simulink model "power_2machinesSVC_PSS"  (Simulink 6.0)
settings: Solver=ode23tb  StartTime=0.0  StopTime=50  MaxStep=1/60  RelTol=1e-4  AbsTol=1e-3
undefined symbols (not defined in the file or in its folder): D1, Delta, find_system, j
libraries: powerlib x18, powerlib2 x8, powerlib_extras x4, simulink_extras x1
settings Model: Creator=sybille  LastModifiedBy=batserve  ExtModeTrigMode=oneshot  ExtModeArmWhenConnect=off  ExtModeAutoUpdateStatusClock=off
settings DataIOCC: LimitDataPoints=off  SignalLoggingName=sigsOut
settings OptimizationCC: BlockReduction=off  BooleanDataType=off
settings DebuggingCC: SolverPrmCheckMsg=none
settings HardwareCC: TargetUnknown=on

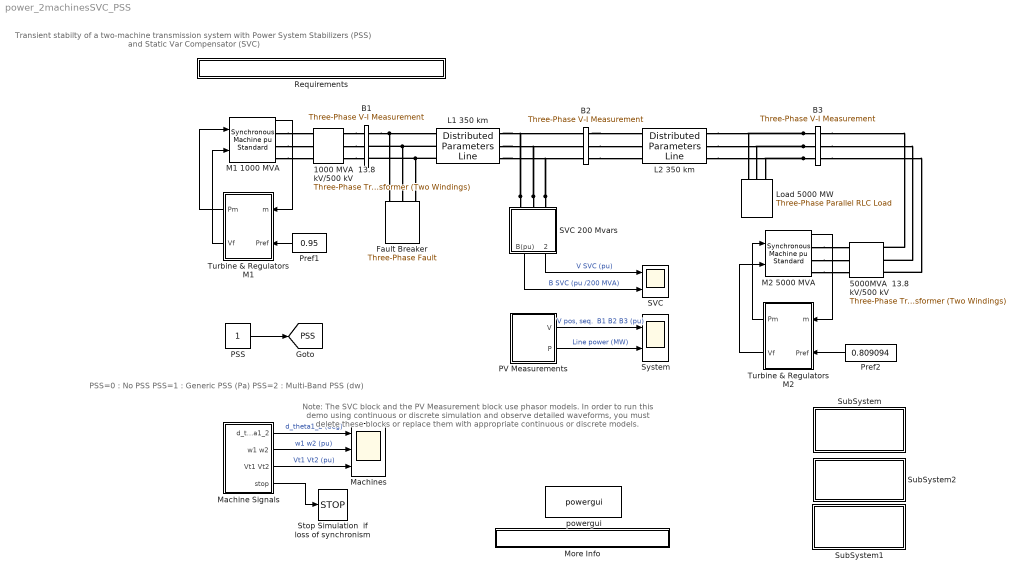
== system power_2machinesSVC_PSS ==
  note: Transient stabilty of a two-machine transmission system
      | with Power System Stabilizers (PSS) and Static Var Compensator (SVC)
  note: Note:
      | The SVC block and the PV Measurement block
      | use phasor models.  In order to run this demo using
      | continuous or discrete simulation and observe detailed
      | waveforms,  you must delete these blocks or replace
      | them with appropriate continuous or discrete models.
  note: PSS=0 : No PSS
      | PSS=1 : Generic PSS (Pa)
      | PSS=2 : Multi-Band PSS (dw)
  1000 MVA  13.8 kV/500 kV : powerlib/Elements/Three-Phase Transformer (Two Windings)  NominalPower=[ 1000e6 60 ]  Winding1Connection=Delta (D1)  Winding1="[ 13.8e3 0.002  0.0]"  Winding2Connection=Yg  Winding2=[ 500e3 0.002 0.12]  SetSaturation=off  Rm=500  Lm=500  Saturation="[ 0,0  ;  0.005,1.2  ;  1.0,1.4 ]"  Hysteresis=off  DataFile='hysteresis'  SetInitialFlux=off  InitialFluxes=[ 0.8 , -0.8 , 0.7 ]  Measurements=None  TransfoNumber=0
  5000MVA  13.8 kV/500 kV : powerlib/Elements/Three-Phase Transformer (Two Windings)  NominalPower=[ 5000e6 60 ]  Winding1Connection=Delta (D1)  Winding1="[ 13.8e3 0.002  0.0]"  Winding2Connection=Yg  Winding2=[ 500e3 0.002 0.12]  SetSaturation=off  Rm=500  Lm=500  Saturation="[ 0,0  ;  0.005,1.2  ;  1.0,1.4 ]"  Hysteresis=off  DataFile='hysteresis'  SetInitialFlux=off  InitialFluxes=[ 0.8 , -0.8 , 0.7 ]  Measurements=None  TransfoNumber=0
  B1 : powerlib/Measurements/Three-Phase V-I Measurement  VoltageMeasurement=phase-to-ground  SetLabelV=on  LabelV=Vabc_B1  Vpu=on  Vbase=500e3  CurrentMeasurement=yes  SetLabelI=on  LabelI=Iabc_B1  Ipu=on  Pbase=100e6  OutputType=Complex  PhasorSimulation=on  PSBequivalent=0
  B2 : powerlib/Measurements/Three-Phase V-I Measurement  VoltageMeasurement=phase-to-ground  SetLabelV=on  LabelV=Vabc_B2  Vpu=on  Vbase=500e3  CurrentMeasurement=no  SetLabelI=on  LabelI=Iabc_B2  Ipu=on  Pbase=100e6  OutputType=Complex  PhasorSimulation=on  PSBequivalent=0
  B3 : powerlib/Measurements/Three-Phase V-I Measurement  VoltageMeasurement=phase-to-ground  SetLabelV=on  LabelV=Vabc_B3  Vpu=on  Vbase=500e3  CurrentMeasurement=no  SetLabelI=off  LabelI=I1  Ipu=off  Pbase=0  OutputType=Complex  PhasorSimulation=on  PSBequivalent=0
  Fault Breaker : powerlib/Elements/Three-Phase Fault  Orientation=down  FaultA=on  FaultB=off  FaultC=off  FaultResistance=0.001  GroundFault=on  GroundResistance=0.001  External=off  SwitchStatus=[1 0]  SwitchTimes=[ 0.1 0.2]  InitialStates=[0 0 1]  SnubberResistance=1e6  SnubberCapacitance=inf  Measurements=None
  L1 350 km : powerlib/Elements/Distributed Parameters Line  Phases=3  Frequency=60  Resistance="[0.01755  0.2758]"  Inductance="[0.8737e-3  3.220e-3]"  Capacitance="[13.33e-9  8.297e-9]"  Length=350  x1=[0 -2.08119625850685e-008 487443.70964158 -112421.385718226;0.000361814960995258 -1.32408804911861e-008 498203.083338567 -45095.3864412803;0.000723629921990516 -5.4238303493389e-009 499707.631423288 23068.3233023193;0.00108544488298577 2.49397509835117e-009 491929.404791019 90803.5063738243;0.00144725984398103 1.03654514377148e-008 475012.894982382 156851.886122394;0.00180907480497629 1.80443748831749e-008 449272.350048993 219986.520650259]  x2=[0 -2.35529805500378e-008 400923.037995999 -306678.651465529;0.000361814960995258 -1.81656675870373e-008 438900.84018104 -249313.294277769;0.000723629921990516 -1.2440901703188e-008 468725.439640532 -187316.590680232;0.00108544488298577 -6.48502850673286e-009 489842.802334574 -121840.216966217;0.00144725984398103 -4.08686750512464e-010 501860.643438643 -54100.489213872;0.00180907480497629 5.67524693906307e-009 504555.714588018 14644.2315021005]  x3=[0 -2.28639731612497e-011 13.1153359399388 -184.480419316447;0.000361814960995258 -1.5497855368557e-011 38.0787449775036 -180.983668896994;0.000723629921990516 -7.84384303326341e-012 62.3347875693628 -174.124891323704;0.00108544488298577 -4.41202400649915e-014 85.4328734808534 -164.031498072894;0.00144725984398103 7.75642214887949e-012 106.943923157398 -150.890988173566;0.00180907480497629 1.54128780462632e-011 126.468338482985 -134.947465148244]  x4=[0 -8.91581395814244e-011 3023.50620810601 -2208.10451815775;0.000361814960995258 -8.08885983149858e-011 3295.677846705 -1776.46366568912;0.000723629921990516 -7.11164371401972e-011 3506.62761662129 -1311.82249270399;0.00108544488298577 -6.00231877467494e-011 3652.43682806992 -822.812364948711;0.00144725984398103 -4.7814922903044e-011 3730.39686910176 -318.517335907422;0.00180907480497629 -3.47184283635963e-011 3739.05952189439 191.694602315866]  x5=0.00180907480497629  Measurements=None
      settings: AttributesFormatString=\n
  L2 350 km : powerlib/Elements/Distributed Parameters Line  Phases=3  Frequency=60  Resistance="[0.01755  0.2758]"  Inductance="[0.8737e-3  3.220e-3]"  Capacitance="[13.33e-9  8.297e-9]"  Length=350  x1=[0 -2.35529805500378e-008 400923.037995999 -306678.651465529;0.000361814960995258 -1.81656675870373e-008 438900.84018104 -249313.294277769;0.000723629921990516 -1.2440901703188e-008 468725.439640532 -187316.590680232;0.00108544488298577 -6.48502850673286e-009 489842.802334574 -121840.216966217;0.00144725984398103 -4.08686750512464e-010 501860.643438643 -54100.489213872;0.00180907480497629 5.67524693906307e-009 504555.714588018 14644.2315021005]  x2=[0 -1.22208025570452e-008 237673.529594385 -435607.401325092;0.000361814960995258 -1.12033805949038e-008 294699.1687201 -399242.932774381;0.000723629921990516 -9.97784002181595e-009 346250.354744666 -355461.963115335;0.00108544488298577 -8.56694698408616e-009 391369.451610182 -305077.785667245;0.00144725984398103 -6.9969108117215e-009 429218.308395391 -249026.357656179;0.00180907480497629 -5.29689714312553e-009 459093.829152304 -188348.913488164]  x3=[0 2.19231358823738e-011 52.7160632692662 -144.994726298769;0.000361814960995258 2.8947525098237e-011 71.9423984147416 -136.479806556214;0.000723629921990516 3.54341731686708e-011 89.8323019448307 -125.429581731223;0.00108544488298577 4.12625814482279e-011 106.053443645353 -112.049325350098;0.00144725984398103 4.63244790248479e-011 120.30449290899 -96.5875945647238;0.00180907480497629 5.05258340049004e-011 132.320716376721 -79.3316128525696]  x4=[0 -9.73737691565742e-011 1740.3123490764 -3266.29894983194;0.000361814960995258 -9.76379763309758e-011 2168.29428893824 -2999.31609805074;0.000723629921990516 -9.60884202544106e-011 2555.99710128903 -2676.61671545742;0.00108544488298577 -9.275388611859e-011 2896.21865904908 -2304.19539865519;0.00144725984398103 -8.76963176026223e-011 3182.63886647449 -1888.97039937023;0.00180907480497629 -8.10096661817247e-011 3409.93706385801 -1438.65510815903]  x5=0.00180907480497629  Measurements=None
      settings: AttributesFormatString=\n
  Load 5000 MW : powerlib/Elements/Three-Phase Parallel RLC Load  Orientation=down  PhysicalDomain=powersysdomain  SubClassName=unknown  LeftPortType=p1  RightPortType=p1  LConnTagsString=A|B|C  Configuration=Y (grounded)  NominalVoltage=500e3  NominalFrequency=60  ActivePower=5000e6  InductivePower=0  CapacitivePower=0  Measurements=None
  M1 1000 MVA : powerlib/Machines/Synchronous Machine pu Standard  PresetModel=No  ShowDetailedParameters=on  RotorType=Salient-pole  NominalParameters="[1000E6  13800   60 ]"  Reactances1=[ 31 32 33 34 35 36 37 ]  Reactances2=[ 1.305, 0.296, 0.252, 0.474, 0.243, 0.18 ]  dAxisTimeConstants=Short-circuit  qAxisTimeConstants=Open-circuit  TimeConstants1=[]  TimeConstants2=[]  TimeConstants3=[]  TimeConstants4=[]  TimeConstants5=[ 1.01, 0.053, 0.1 ]  TimeConstants6=[]  TimeConstants7=[]  TimeConstants8=[]  StatorResistance=2.8544e-3  Mechanical="[ 3.7 0  32]"  InitialConditions=[0 -16.6861 0.950218 0.950218 0.950218 48.1093 -71.8907 168.109 1.44424]  SetSaturation=off  Saturation=[0.6404,0.7127,0.8441,0.9214,0.9956,1.082,1.19,1.316,1.457;0.7,0.7698,0.8872,0.9466,0.9969,1.046,1.1,1.151,1.201]  Units=0.5  LoadFlowParameters=[1 950000000 0 0]
      settings: AttributesFormatString=\n\n
  M2 5000 MVA : powerlib/Machines/Synchronous Machine pu Standard  PresetModel=No  ShowDetailedParameters=on  RotorType=Salient-pole  NominalParameters="[5000E6  13800   60 ]"  Reactances1=[ 31 32 33 34 35 36 37 ]  Reactances2=[ 1.305, 0.296, 0.252, 0.474, 0.243, 0.18 ]  dAxisTimeConstants=Short-circuit  qAxisTimeConstants=Open-circuit  TimeConstants1=[]  TimeConstants2=[]  TimeConstants3=[]  TimeConstants4=[]  TimeConstants5=[ 1.01, 0.053, 0.1 ]  TimeConstants6=[]  TimeConstants7=[]  TimeConstants8=[]  StatorResistance=2.8544e-3  Mechanical="[ 3.7 0  32]"  InitialConditions=[0 -69.7487 0.812764 0.812764 0.812764 -5.44703 -125.447 114.553 1.40021]  SetSaturation=off  Saturation=[0.6404,0.7127,0.8441,0.9214,0.9956,1.082,1.19,1.316,1.457;0.7,0.7698,0.8872,0.9466,0.9969,1.046,1.1,1.151,1.201]  Units=0.5  LoadFlowParameters=[2 4000000000 0 0]
      settings: AttributesFormatString=\n\n
  Machine Signals : Subsystem
  Machines : Scope  NumInputPorts=3
      settings: TimeRange=50  YMin=30~0.995~0  YMax=70~1.005~1.5  SaveName=mach
  More Info : Subsystem
      settings: OpenFcn=web(which('psb2machines.html'));
      mask Display: disp('? : Double click here for more info')
  PSS : Constant
  PV Measurements : Subsystem
  "Pref1 " : Constant  Orientation=left  Value=0.95
  Pref2 : Constant  Orientation=left  Value=0.809094
  Requirements : Subsystem  Description=|  LoadFcn=|  InitFcn=|
      LoadFcn=|
      | Toolboxes = ver;                                                                                                                              
      | installedtoolboxes = {Toolboxes.Name};                                                                                                        
      | k = strcmp('Control System Toolbox',installedtoolboxes);                                                                                      
      | if ~any(k)                                                                                                                                    
      |     H = warndlg(['You need to install the Control System Toolbox in order to run the power_2machinesSVC_PSS demo'],'SimPowerSystems warning');
      |     uiwait(H);                                                                                                                                
      | end
      InitFcn=|
      | Toolboxes = ver;                                                                                               
      | installedtoolboxes = {Toolboxes.Name};                                                                         
      | k = strcmp('Control System Toolbox',installedtoolboxes);                                                       
      | if ~any(k)                                                                                                     
      |     error(['You need to install the Control System Toolbox in order to run the power_2machinesSVC_PSS demo.']);
      | end
      Description=|
      | This block is used to popup errors and warnings if the
      | Control System Toolbox is not installed.
      settings: OpenFcn=|
      | Toolboxes = ver;
      | installedtoolboxes = {Toolboxes.Name};
      | k = strcmp('Control System Toolbox',installedtoolboxes);
      | if ~any(k)
      |     warndlg(['You need to install the Control System Toolbox in order to run the power_2machinesSVC_PSS demo.'],'SimPowerSystems warning');
      |                                                                                                                                                         end
      mask Display: disp('This demo requires the Control System Toolbox')
  SVC : Scope  NumInputPorts=2
      settings: TimeRange=10  YMin=0.5~-1  YMax=1.1~1  SaveName=svc
  SVC 200 Mvars : Subsystem  Orientation=down  AncestorBlock=powerlib/Phasor Elements/Static Var Compensator  LoadFcn=find_system(gcs,'FollowLinks', 'on', 'LookUnderMasks', 'all');  mask(Static Var Compensator (Phasor Type)){mode=Var control (Fixed susceptance Bref), Vnom=500e3, Qnom=[200e6 -200e6], Pbase=200e6, Vref=1.009, Xs=0.03, Kp_Ki=[0  333], Bref=0.0, Tm=8e-3, Td=4e-3}
      mask prompts: mode "Mode of operation"; Vnom "Nominal voltage (Vrms Ph-Ph):"; Qnom "Reactive power limits [Qc(var>0)  Ql(var<0)]:"; Pbase "Three-phase base power Pbase (VA):"; Vref "Reference voltage Vref  (pu):"; Xs "Droop Xs (pu/Pbase):"; Kp_Ki "Voltage regulator [Kp(puB/puV)  Ki(puB/puV/s)]:"; Bref "Bref  for var control mode (pu/Pbase):"; Tm "Time constant of voltage measurement system Tm (s):"; Td "Average time delay due to thyristor valves firing Td (s):"
      mask help:
      | This block implements a  phasor model of a three-phase, three-wire Static Var Compensator (SVC).
      |
      | The B output signal (SVC susceptance in pu/Pbase)  is the output of the voltage regulator or the reference susceptance Bref in var control mode.
      | The Vm output is the measured positive-sequence voltage (pu).
      mask init:
      | Qc_nom=Qnom(1);
      | Ql_nom=Qnom(2);
      | Bmax=Qc_nom/Pbase;
      | Bmin=Ql_nom/Pbase;
      | Vbase=Vnom/sqrt(3)*sqrt(2);
      | Ibase=Pbase/Vnom/sqrt(3)*sqrt(2);
      | Kp=Kp_Ki(1);
      | Ki=Kp_Ki(2);;
      settings: CloseFcn=%3phaseVImeasurement
      mask Help: web(psbhelp)
      mask StyleString: popup(Voltage regulation|Var control (Fixed susceptance Bref)),edit,edit,edit,edit,edit,edit,edit,edit,edit
      mask CallbackString: powericon('psbcallbacks',gcb,'SVCblock');|||||||||
  Stop Simulation  if loss of synchronism : Stop
  SubSystem : Subsystem
      settings: OpenFcn=openfig('psb2macSVC_PhasorVsDet.fig');
      mask Display: disp('Show comparison\nDetailed vs Phasor\n simulation')
  SubSystem1 : Subsystem
      settings: OpenFcn=openfig('psb2macSVC_3phfault.fig');
      mask Display: disp('Show impact of SVC\nfor 3-phase fault')
  SubSystem2 : Subsystem
      settings: OpenFcn=openfig('psb2macSVC_1phfault.fig');
      mask Display: disp('Show impact of PSS\nfor 1-phase fault')
  System : Scope  NumInputPorts=2
      settings: TimeRange=50  YMin=0~0  YMax=1.5~1500  SaveName=mach1
  Turbine & Regulators M1 : Subsystem  Orientation=left
  Turbine & Regulators M2 : Subsystem  Orientation=left
  powergui : powerlib/powergui  Priority=2  Frange=[0:2:500]  Ylog=off  Xlog=off  save=off  variable=ZData  ZoomFFT=on  StartTime=0.0  cycles=1  DisplayStyle=off  fundamental=60  FreqAxis=off  MaxFrequency=1000  frequencyindice=60  frequencyindicesteady=1  RmsSteady=1  display=off  Ts=0  methode=on  frequency=60  echomessages=on
  tag scope: PSS=global
  wires:
  Pref2/1 -> Turbine & Regulators M2/2(Pref)
  Machine Signals/2(w1 w2) -> Machines/2  "w1 w2 (pu)"
  Machine Signals/1(d_theta1_2) -> Machines/1  "d_theta1_2 (deg)"
  Machine Signals/4(stop) -> Stop Simulation  if loss of synchronism/1
  Machine Signals/3(Vt1 Vt2) -> Machines/3  "Vt1 Vt2 (pu)"
  "Pref1 "/1 -> Turbine & Regulators M1/2(Pref)
  PV Measurements/1(V) -> System/1  "V pos, seq.  B1 B2 B3 (pu)"
  PV Measurements/2(P) -> System/2  "Line power (MW)"
  Turbine & Regulators M1/1(Pm) -> M1 1000 MVA/1
  Turbine & Regulators M1/2(Vf) -> M1 1000 MVA/2
  SVC 200 Mvars/2(Vm(pu)) -> SVC/1  "V SVC (pu)"
  SVC 200 Mvars/1(B(pu)) -> SVC/2  "B SVC (pu /200 MVA)"
  Turbine & Regulators M2/1(Pm) -> M2 5000 MVA/1
  Turbine & Regulators M2/2(Vf) -> M2 5000 MVA/2
  M1 1000 MVA/1 -> Turbine & Regulators M1/1(m)
  M2 5000 MVA/1 -> Turbine & Regulators M2/1(m)
  PSS/1 -> [PSS]
  connections:
  B3/LConn3 -- L2 350 km/RConn3 -- Load 5000 MW/LConn3
  B3/LConn2 -- L2 350 km/RConn2 -- Load 5000 MW/LConn2
  B3/LConn1 -- L2 350 km/RConn1 -- Load 5000 MW/LConn1
  L1 350 km/LConn2 -- B1/RConn2 -- Fault Breaker/LConn2
  1000 MVA  13.8 kV/500 kV/RConn2 -- B1/LConn2
  1000 MVA  13.8 kV/500 kV/RConn1 -- B1/LConn1
  L1 350 km/LConn3 -- B1/RConn3 -- Fault Breaker/LConn3
  1000 MVA  13.8 kV/500 kV/RConn3 -- B1/LConn3
  M1 1000 MVA/RConn1 -- 1000 MVA  13.8 kV/500 kV/LConn1
  M1 1000 MVA/RConn2 -- 1000 MVA  13.8 kV/500 kV/LConn2
  M1 1000 MVA/RConn3 -- 1000 MVA  13.8 kV/500 kV/LConn3
  M2 5000 MVA/RConn1 -- 5000MVA  13.8 kV/500 kV/LConn1
  M2 5000 MVA/RConn2 -- 5000MVA  13.8 kV/500 kV/LConn2
  M2 5000 MVA/RConn3 -- 5000MVA  13.8 kV/500 kV/LConn3
  SVC 200 Mvars/LConn2 -- L1 350 km/RConn2 -- B2/LConn2
  SVC 200 Mvars/LConn1 -- L1 350 km/RConn1 -- B2/LConn1
  SVC 200 Mvars/LConn3 -- L1 350 km/RConn3 -- B2/LConn3
  B2/RConn1 -- L2 350 km/LConn1
  B2/RConn2 -- L2 350 km/LConn2
  B2/RConn3 -- L2 350 km/LConn3
  B1/RConn1 -- L1 350 km/LConn1 -- Fault Breaker/LConn1
  B3/RConn1 -- 5000MVA  13.8 kV/500 kV/RConn1
  B3/RConn2 -- 5000MVA  13.8 kV/500 kV/RConn2
  B3/RConn3 -- 5000MVA  13.8 kV/500 kV/RConn3

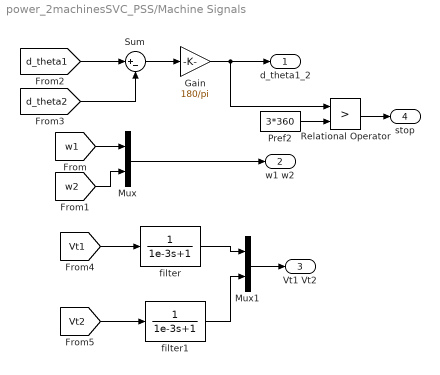
== system power_2machinesSVC_PSS/Machine Signals ==
  " filter" : TransferFcn  Denominator=[1e-3 1]
  " filter1" : TransferFcn  Denominator=[1e-3 1]
  Gain : Gain  Gain=180/pi  SaturateOnIntegerOverflow=on
  Mux : Mux  Inputs=2
  Mux1 : Mux  Inputs=2
  Pref2 : Constant  Value=3*360
  Relational Operator : RelationalOperator  Operator=>  InputSameDT=on
  Sum : Sum  Inputs=|+-  SaturateOnIntegerOverflow=on  InputSameDT=on
  d_theta1_2 : Outport
  w1 w2 : Outport  Port=2
  Vt1 Vt2 : Outport  Port=3
  stop : Outport  Port=4
  wires:
  Sum/1 -> Gain/1
  [d_theta1] -> Sum/1
  [w1] -> Mux/1
  Mux/1 -> w1 w2/1
  Gain/1 -> d_theta1_2/1, Relational Operator/1
  [w2] -> Mux/2
  [d_theta2] -> Sum/2
  [Vt1] -> " filter"/1
  Mux1/1 -> Vt1 Vt2/1
  [Vt2] -> " filter1"/1
  Pref2/1 -> Relational Operator/2
  Relational Operator/1 -> stop/1
  " filter"/1 -> Mux1/1
  " filter1"/1 -> Mux1/2

== system power_2machinesSVC_PSS/More Info ==

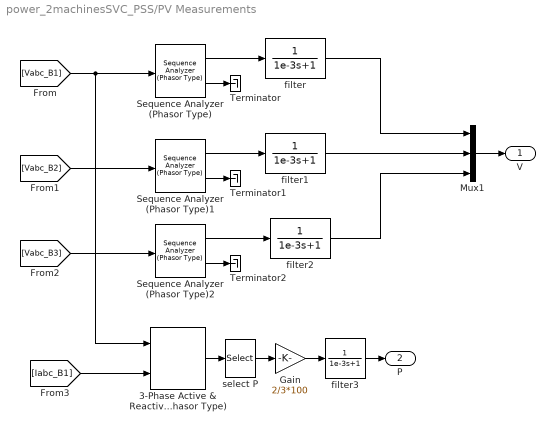
== system power_2machinesSVC_PSS/PV Measurements ==
   filter{,1..3} (4 alike) : TransferFcn  Denominator=[1e-3 1]
  3-Phase Active & Reactive Power (Phasor Type) : powerlib_extras/Phasor Library/3-Phase Active & Reactive Power (Phasor Type)
  Gain : Gain  Gain=2/3*100  SaturateOnIntegerOverflow=on
  Mux1 : Mux  Inputs=3
  Sequence Analyzer (Phasor Type) : powerlib_extras/Phasor Library/Sequence Analyzer (Phasor Type)  seq=Positive
  Sequence Analyzer (Phasor Type)1 : powerlib_extras/Phasor Library/Sequence Analyzer (Phasor Type)  seq=Positive
  Sequence Analyzer (Phasor Type)2 : powerlib_extras/Phasor Library/Sequence Analyzer (Phasor Type)  seq=Positive
  Terminator : Terminator
  Terminator1 : Terminator
  Terminator2 : Terminator
  select P : Selector  InputPortWidth=2
  V : Outport
  P : Outport  Port=2
  wires:
  " filter3"/1 -> P/1
  Gain/1 -> " filter3"/1
  3-Phase Active & Reactive Power (Phasor Type)/1 -> select P/1
  [Iabc_B1] -> 3-Phase Active & Reactive Power (Phasor Type)/2
  Sequence Analyzer (Phasor Type)2/2 -> Terminator2/1
  Sequence Analyzer (Phasor Type)1/2 -> Terminator1/1
  Sequence Analyzer (Phasor Type)/2 -> Terminator/1
  " filter2"/1 -> Mux1/3
  " filter1"/1 -> Mux1/2
  " filter"/1 -> Mux1/1
  Mux1/1 -> V/1
  Sequence Analyzer (Phasor Type)2/1 -> " filter2"/1
  Sequence Analyzer (Phasor Type)1/1 -> " filter1"/1
  [Vabc_B3] -> Sequence Analyzer (Phasor Type)2/1
  [Vabc_B2] -> Sequence Analyzer (Phasor Type)1/1
  Sequence Analyzer (Phasor Type)/1 -> " filter"/1
  [Vabc_B1] -> 3-Phase Active & Reactive Power (Phasor Type)/1, Sequence Analyzer (Phasor Type)/1
  select P/1 -> Gain/1

== system power_2machinesSVC_PSS/Requirements ==

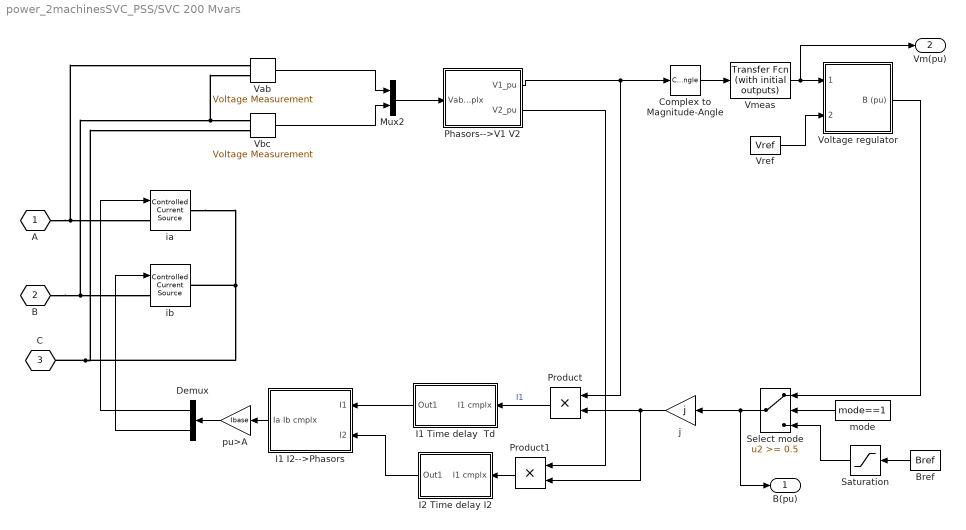
== system power_2machinesSVC_PSS/SVC 200 Mvars ==
  Bref : Constant  Orientation=left  Value=Bref
  Complex to Magnitude-Angle : ComplexToMagnitudeAngle  Output=Magnitude
  Demux : Demux  Orientation=left  Outputs=2
  I1 I2-->Phasors : Subsystem  Orientation=left
  I1 Time delay  Td : Subsystem  Orientation=left
  I2 Time delay I2 : Subsystem  Orientation=left
  Mux2 : Mux  Inputs=2
  Phasors-->V1 V2 : Subsystem
  Product : Product  Orientation=left  SaturateOnIntegerOverflow=on  InputSameDT=on
  Product1 : Product  Orientation=left  SaturateOnIntegerOverflow=on  InputSameDT=on
  Saturation : Saturate  Orientation=left  UpperLimit=Bmax  LowerLimit=Bmin
  Select mode : Switch  Orientation=left  Threshold=0.5  InputSameDT=on
  Vab : powerlib/Measurements/Voltage Measurement  PhasorSimulation=on  OutputType=Complex  PSBequivalent=0
  Vbc : powerlib/Measurements/Voltage Measurement  PhasorSimulation=on  OutputType=Complex  PSBequivalent=0
  Vmeas : simulink_extras/Additional Linear/Transfer Fcn (with initial outputs)  N=[1]  D="[Tm  1]"  Y0=Vref  U0=Vref
  Voltage regulator : Subsystem
  Vref : Constant  Value=Vref
  ia : powerlib/Electrical Sources/Controlled Current Source  Description=source block  Initialize=off  Amplitude=0  Phase=0  Frequency=0  Measurements=None
  ib : powerlib/Electrical Sources/Controlled Current Source  Description=source block  Initialize=off  Amplitude=0  Phase=0  Frequency=0  Measurements=None
  j : Gain  Orientation=left  Gain=j  SaturateOnIntegerOverflow=on
  mode : Constant  Orientation=left  Value=mode==1
  pu>A : Gain  Orientation=left  Gain=Ibase  SaturateOnIntegerOverflow=on
  A : PMIOPort  Port=1  Side=Left
  B : PMIOPort  Port=2  Side=Left
  C : PMIOPort  Port=3  Side=Left
  B(pu) : Outport
  Vm(pu) : Outport  Port=2
  wires:
  Product1/1 -> I2 Time delay I2/1(I1 cmplx)
  Phasors-->V1 V2/2(V2_pu) -> Product1/1
  j/1 -> Product1/2, Product/2
  Product/1 -> I1 Time delay  Td/1(I1 cmplx)  "I1"
  pu>A/1 -> Demux/1
  I1 Time delay  Td/1(Out1) -> I1 I2-->Phasors/1(I1)
  Vbc/1 -> Mux2/2
  Vab/1 -> Mux2/1
  Complex to Magnitude-Angle/1 -> Vmeas/1
  I2 Time delay I2/1(Out1) -> I1 I2-->Phasors/2(I2)
  I1 I2-->Phasors/1(Ia Ib cmplx) -> pu>A/1
  Vmeas/1 -> Vm(pu)/1, Voltage regulator/1(V1meas (pu))
  Vref/1 -> Voltage regulator/2(Vref (pu))
  Phasors-->V1 V2/1(V1_pu) -> Product/1, Complex to Magnitude-Angle/1
  Mux2/1 -> Phasors-->V1 V2/1(Vab Vbc cmplx)
  Select mode/1 -> j/1, B(pu)/1
  Bref/1 -> Saturation/1
  Voltage regulator/1(B (pu)) -> Select mode/1
  mode/1 -> Select mode/2
  Demux/1 -> ia/1
  Demux/2 -> ib/1
  Saturation/1 -> Select mode/3
  connections:
  A/RConn1 -- ia/LConn1 -- Vab/LConn1
  B/RConn1 -- ib/LConn1 -- Vbc/LConn1 -- Vab/LConn2
  ia/RConn1 -- ib/RConn1 -- C/RConn1 -- Vbc/LConn2

== system power_2machinesSVC_PSS/SubSystem ==

== system power_2machinesSVC_PSS/SubSystem1 ==

== system power_2machinesSVC_PSS/SubSystem2 ==

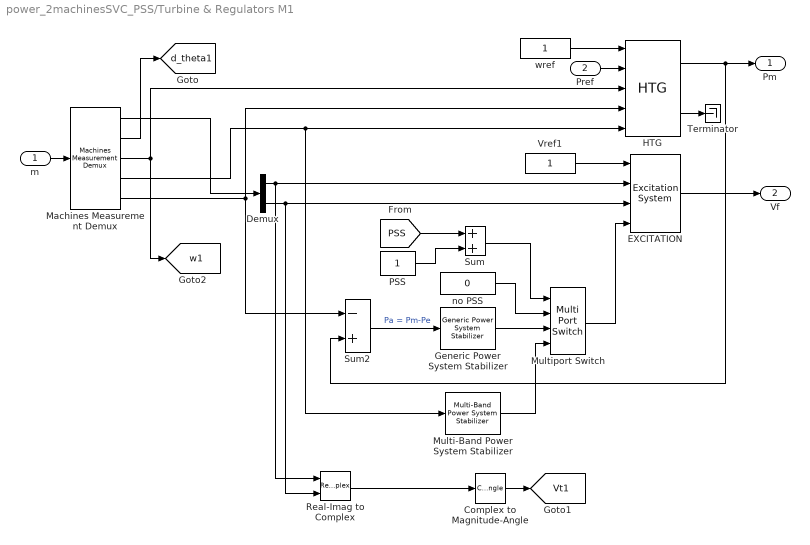
== system power_2machinesSVC_PSS/Turbine & Regulators M1 ==
  m : Inport  Port=1  LatchInput=off
  Pref : Inport  Port=2  LatchInput=off
  Complex to Magnitude-Angle : ComplexToMagnitudeAngle  Output=Magnitude
  Demux : Demux  Outputs=2
  EXCITATION : powerlib2/Machines/Excitation System  tr=20e-3  reg=[ 200, 0.001 ]  exc=[ 1, 0 ]  tgr=[ 0, 0 ]  damp=[ 0.001, 0.1 ]  sat=[ 0, 0 ]  lim="[ 0,  7, 0 ]"  v0=[1,1.44424]
  Generic Power System Stabilizer : powerlib2/Machines/Generic Power System Stabilizer  Tsensor=15e-3  K=2  Twashout=0.7  Tleadlag1="[60e-3  0.5]"  Tleadlag2=[0 0]  VSlimits=[-0.15 0.15]  Vinit=0  Plot_On=off  MagdB_On=on  FreqRange=logspace(-2,2,500)
  HTG : powerlib2/Machines/HTG  sm="[ 10/3  0.07 ]"  gate="[  0.01  0.97518  -0.1  0.1 ]"  reg="[  0.05  1.163  0.105  0  0.01  ]"  hyd="[  0  2.67  ]"  dref=0  po=0.952577
  Machines Measurement Demux : powerlib2/Machines/Machines Measurement Demux  machType=Synchronous  ssm1=on  ssm2=on  ssm3=on  ssm4=on  ssm5=on  ssm6=on  sm1=off  sm2=off  sm3=off  sm4=off  sm5=off  sm6=on  sm7=on  sm8=on  sm9=off  sm10=on  sm11=off  sm115=off  sm12=off  sm13=on  sm14=off  asm1=on  asm2=on  asm3=on  asm4=on  asm5=on  asm6=on  asm7=on  asm8=on  asm9=on  asm10=on  asm11=on  pmsm1=on  pmsm2=on  pmsm3=on  pmsm4=on  pmsm5=on  pmsm6=on  lastType=2
  Multi-Band Power System Stabilizer : powerlib/Machines/Multi-Band Power System Stabilizer  OperationMode=Simplified settings  Kg=1.0  GL=[0.025 5]  GI=[0.8 25]  GH=[12.0 145]  GLd=[66 66 9.4]  TcLF=[1.667 2 0 0 0 0 2 2.4 0 0 0 0 1 1]  GId=[66 66 47.6]  TcIF=[1 1 0.25 0.3 0 0 1 1 0.3 0.36 0 0 0 0]  GHd=[66 66 233]  TcHF="[0.01 0.012 0 0 0 0  0.012 0.0144 0 0 0 0 1 1]"  LIM=[.075 .15 .15 .15]  Plot_On=off  MagdB_On=off  FreqRange=logspace(-2,2,500)
  Multiport Switch : MultiPortSwitch  Inputs=3  SaturateOnIntegerOverflow=on
  PSS : Constant
  Real-Imag to Complex : RealImagToComplex
  Sum : Sum  SaturateOnIntegerOverflow=on
  Sum2 : Sum  Inputs=-+  SaturateOnIntegerOverflow=on  InputSameDT=on
  Terminator : Terminator
  Vref1 : Constant
  no PSS : Constant  Value=0
  wref : Constant
  Pm : Outport  InitialOutput=0
  Vf : Outport  Port=2  InitialOutput=0
  tag scope: Vt1=global, d_theta1=global, w1=global
  wires:
  Real-Imag to Complex/1 -> Complex to Magnitude-Angle/1
  HTG/2 -> Terminator/1
  Vref1/1 -> EXCITATION/1
  m/1 -> Machines Measurement Demux/1
  Machines Measurement Demux/1 -> Demux/1
  Machines Measurement Demux/4 -> HTG/5, Multi-Band Power System Stabilizer/1
  Machines Measurement Demux/5 -> HTG/4, Sum2/1
  Machines Measurement Demux/3 -> [w1], HTG/3
  Pref/1 -> HTG/2
  wref/1 -> HTG/1
  HTG/1 -> Pm/1, Sum2/2
  Demux/2 -> Real-Imag to Complex/2, EXCITATION/3
  EXCITATION/1 -> Vf/1
  Demux/1 -> Real-Imag to Complex/1, EXCITATION/2
  Complex to Magnitude-Angle/1 -> [Vt1]
  Machines Measurement Demux/2 -> [d_theta1]
  Sum2/1 -> Generic Power System Stabilizer/1  "Pa = Pm-Pe"
  Generic Power System Stabilizer/1 -> Multiport Switch/3
  Multi-Band Power System Stabilizer/1 -> Multiport Switch/4
  no PSS/1 -> Multiport Switch/2
  Multiport Switch/1 -> EXCITATION/4
  [PSS] -> Sum/1
  PSS/1 -> Sum/2
  Sum/1 -> Multiport Switch/1

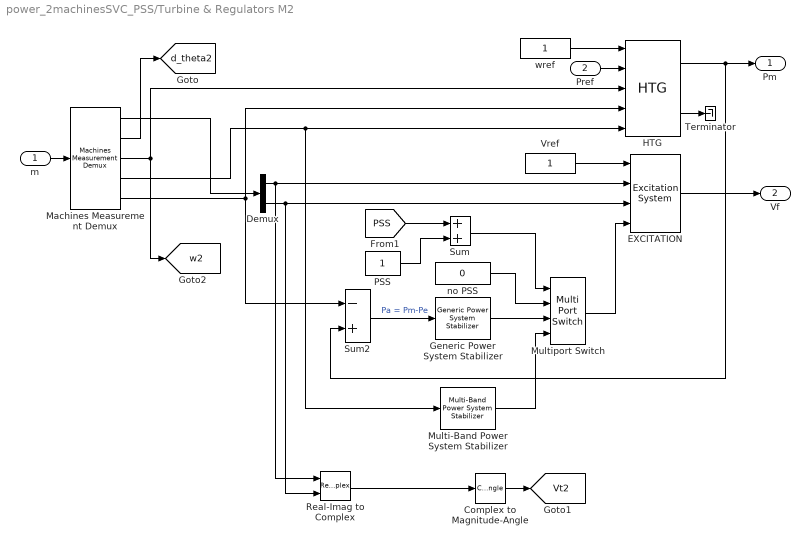
== system power_2machinesSVC_PSS/Turbine & Regulators M2 ==
  m : Inport  Port=1  LatchInput=off
  Pref : Inport  Port=2  LatchInput=off
  Complex to Magnitude-Angle : ComplexToMagnitudeAngle  Output=Magnitude
  Demux : Demux  Outputs=2
  EXCITATION : powerlib2/Machines/Excitation System  tr=20e-3  reg=[ 200, 0.001 ]  exc=[ 1, 0 ]  tgr=[ 0, 0 ]  damp=[ 0.001, 0.1 ]  sat=[ 0, 0 ]  lim="[ 0,  7, 0 ]"  v0=[1,1.40021]
  Generic Power System Stabilizer : powerlib2/Machines/Generic Power System Stabilizer  Tsensor=15e-3  K=2  Twashout=0.7  Tleadlag1="[60e-3  0.5]"  Tleadlag2=[0 0]  VSlimits=[-0.15 0.15]  Vinit=0  Plot_On=off  MagdB_On=on  FreqRange=logspace(-2,2,500)
  HTG : powerlib2/Machines/HTG  sm="[ 10/3  0.07 ]"  gate="[  0.01  0.97518  -0.1  0.1 ]"  reg="[  0.05  1.163  0.105  0  0.01  ]"  hyd="[  0  2.67  ]"  dref=0  po=0.810979
  Machines Measurement Demux : powerlib2/Machines/Machines Measurement Demux  machType=Synchronous  ssm1=on  ssm2=on  ssm3=on  ssm4=on  ssm5=on  ssm6=on  sm1=off  sm2=off  sm3=off  sm4=off  sm5=off  sm6=on  sm7=on  sm8=on  sm9=off  sm10=on  sm11=off  sm115=off  sm12=off  sm13=on  sm14=off  asm1=on  asm2=on  asm3=on  asm4=on  asm5=on  asm6=on  asm7=on  asm8=on  asm9=on  asm10=on  asm11=on  pmsm1=on  pmsm2=on  pmsm3=on  pmsm4=on  pmsm5=on  pmsm6=on  lastType=2
  Multi-Band Power System Stabilizer : powerlib/Machines/Multi-Band Power System Stabilizer  OperationMode=Simplified settings  Kg=1.0  GL=[0.025 5]  GI=[0.8 25]  GH=[12.0 145]  GLd=[66 66 9.4]  TcLF=[1.667 2 0 0 0 0 2 2.4 0 0 0 0 1 1]  GId=[66 66 47.6]  TcIF=[1 1 0.25 0.3 0 0 1 1 0.3 0.36 0 0 0 0]  GHd=[66 66 233]  TcHF="[0.01 0.012 0 0 0 0  0.012 0.0144 0 0 0 0 1 1]"  LIM=[.075 .15 .15 .15]  Plot_On=off  MagdB_On=off  FreqRange=logspace(-2,2,500)
  Multiport Switch : MultiPortSwitch  Inputs=3  SaturateOnIntegerOverflow=on
  PSS : Constant
  Real-Imag to Complex : RealImagToComplex
  Sum : Sum  SaturateOnIntegerOverflow=on
  Sum2 : Sum  Inputs=-+  SaturateOnIntegerOverflow=on  InputSameDT=on
  Terminator : Terminator
  Vref : Constant
  no PSS : Constant  Value=0
  wref : Constant
  Pm : Outport  InitialOutput=0
  Vf : Outport  Port=2  InitialOutput=0
  tag scope: Vt2=global, d_theta2=global, w2=global
  wires:
  Multiport Switch/1 -> EXCITATION/4
  Sum/1 -> Multiport Switch/1
  no PSS/1 -> Multiport Switch/2
  Multi-Band Power System Stabilizer/1 -> Multiport Switch/4
  Generic Power System Stabilizer/1 -> Multiport Switch/3
  Sum2/1 -> Generic Power System Stabilizer/1  "Pa = Pm-Pe"
  Machines Measurement Demux/2 -> [d_theta2]
  Complex to Magnitude-Angle/1 -> [Vt2]
  Demux/1 -> EXCITATION/2, Real-Imag to Complex/1
  EXCITATION/1 -> Vf/1
  Demux/2 -> EXCITATION/3, Real-Imag to Complex/2
  HTG/1 -> Sum2/2, Pm/1
  wref/1 -> HTG/1
  Pref/1 -> HTG/2
  Machines Measurement Demux/3 -> HTG/3, [w2]
  Machines Measurement Demux/5 -> HTG/4, Sum2/1
  Machines Measurement Demux/4 -> Multi-Band Power System Stabilizer/1, HTG/5
  Machines Measurement Demux/1 -> Demux/1
  m/1 -> Machines Measurement Demux/1
  Vref/1 -> EXCITATION/1
  HTG/2 -> Terminator/1
  Real-Imag to Complex/1 -> Complex to Magnitude-Angle/1
  [PSS] -> Sum/1
  PSS/1 -> Sum/2

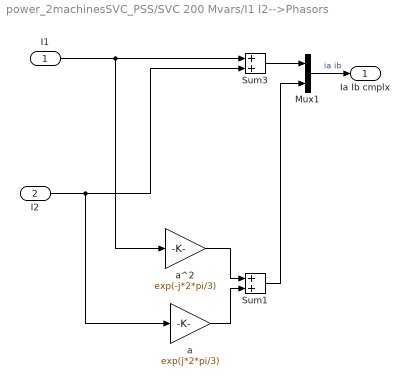
== system power_2machinesSVC_PSS/SVC 200 Mvars/I1 I2-->Phasors ==
  I1 : Inport  Port=1  LatchInput=off
  I2 : Inport  Port=2  LatchInput=off
  Mux1 : Mux  Inputs=2
  Sum1 : Sum  SaturateOnIntegerOverflow=on  InputSameDT=on
  Sum3 : Sum  SaturateOnIntegerOverflow=on  InputSameDT=on
  a : Gain  Gain=exp(j*2*pi/3)  SaturateOnIntegerOverflow=on
  a^2 : Gain  Gain=exp(-j*2*pi/3)  SaturateOnIntegerOverflow=on
  Ia Ib cmplx : Outport
  wires:
  I1/1 -> a^2/1, Sum3/1
  I2/1 -> a/1, Sum3/2
  a^2/1 -> Sum1/1
  a/1 -> Sum1/2
  Sum3/1 -> Mux1/1
  Sum1/1 -> Mux1/2
  Mux1/1 -> Ia Ib cmplx/1  "ia ib"

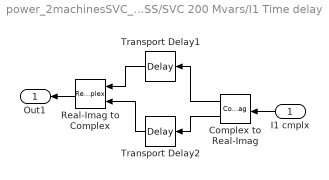
== system power_2machinesSVC_PSS/SVC 200 Mvars/I1 Time delay  Td ==
  I1 cmplx : Inport  Orientation=left  Port=1  LatchInput=off
  Complex to Real-Imag : ComplexToRealImag  Orientation=left
  Real-Imag to Complex : RealImagToComplex  Orientation=left
  Transport Delay1 : TransportDelay  Orientation=left  DelayTime=Td
  Transport Delay2 : TransportDelay  Orientation=left  DelayTime=Td
  Out1 : Outport  Orientation=left
  wires:
  Transport Delay2/1 -> Real-Imag to Complex/2
  Transport Delay1/1 -> Real-Imag to Complex/1
  Complex to Real-Imag/2 -> Transport Delay2/1
  Complex to Real-Imag/1 -> Transport Delay1/1
  Real-Imag to Complex/1 -> Out1/1
  I1 cmplx/1 -> Complex to Real-Imag/1

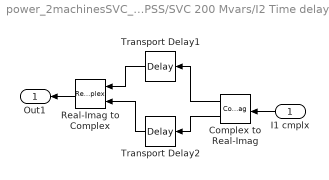
== system power_2machinesSVC_PSS/SVC 200 Mvars/I2 Time delay I2 ==
  I1 cmplx : Inport  Orientation=left  Port=1  LatchInput=off
  Complex to Real-Imag : ComplexToRealImag  Orientation=left
  Real-Imag to Complex : RealImagToComplex  Orientation=left
  Transport Delay1 : TransportDelay  Orientation=left  DelayTime=Td
  Transport Delay2 : TransportDelay  Orientation=left  DelayTime=Td
  Out1 : Outport  Orientation=left
  wires:
  I1 cmplx/1 -> Complex to Real-Imag/1
  Real-Imag to Complex/1 -> Out1/1
  Complex to Real-Imag/1 -> Transport Delay1/1
  Complex to Real-Imag/2 -> Transport Delay2/1
  Transport Delay1/1 -> Real-Imag to Complex/1
  Transport Delay2/1 -> Real-Imag to Complex/2

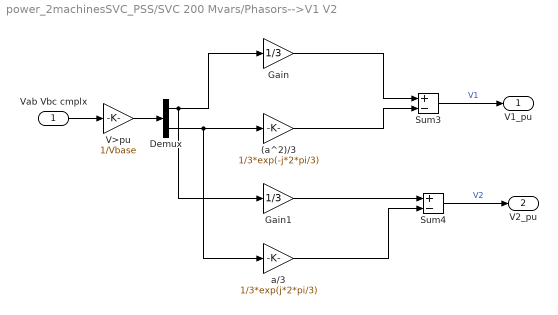
== system power_2machinesSVC_PSS/SVC 200 Mvars/Phasors-->V1 V2 ==
  Vab Vbc cmplx : Inport  Port=1  LatchInput=off
  (a^2)/3 : Gain  Gain=1/3*exp(-j*2*pi/3)  SaturateOnIntegerOverflow=on
  Demux : Demux  Outputs=2
  Gain : Gain  Gain=1/3  SaturateOnIntegerOverflow=on
  Gain1 : Gain  Gain=1/3  SaturateOnIntegerOverflow=on
  Sum3 : Sum  Inputs=+-  SaturateOnIntegerOverflow=on  InputSameDT=on
  Sum4 : Sum  Inputs=+-  SaturateOnIntegerOverflow=on  InputSameDT=on
  V>pu : Gain  Gain=1/Vbase  SaturateOnIntegerOverflow=on
  a/3 : Gain  Gain=1/3*exp(j*2*pi/3)  SaturateOnIntegerOverflow=on
  V1_pu : Outport
  V2_pu : Outport  Port=2
  wires:
  V>pu/1 -> Demux/1
  Sum3/1 -> V1_pu/1  "V1"
  Demux/1 -> Gain1/1, Gain/1
  a/3/1 -> Sum4/2
  Gain1/1 -> Sum4/1
  Vab Vbc cmplx/1 -> V>pu/1
  Gain/1 -> Sum3/1
  Demux/2 -> a/3/1, (a^2)/3/1
  (a^2)/3/1 -> Sum3/2
  Sum4/1 -> V2_pu/1  "V2"

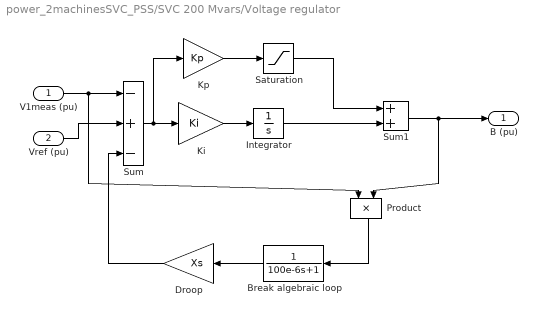
== system power_2machinesSVC_PSS/SVC 200 Mvars/Voltage regulator ==
  V1meas (pu) : Inport  Port=1  LatchInput=off
  Vref (pu) : Inport  Port=2  LatchInput=off
  Break algebraic loop : TransferFcn  Orientation=left  Denominator=[100e-6 1]
  Droop : Gain  Orientation=left  Gain=Xs  SaturateOnIntegerOverflow=on
  Integrator : Integrator  LimitOutput=on  UpperSaturationLimit=Bmax  LowerSaturationLimit=Bmin
  Ki : Gain  Gain=Ki  SaturateOnIntegerOverflow=on
  Kp : Gain  Gain=Kp  SaturateOnIntegerOverflow=on
  Product : Product  Orientation=down  SaturateOnIntegerOverflow=on  InputSameDT=on
  Saturation : Saturate  UpperLimit=Bmax  LowerLimit=Bmin
  Sum : Sum  Inputs=-+-  SaturateOnIntegerOverflow=on  InputSameDT=on
  Sum1 : Sum  SaturateOnIntegerOverflow=on
  B (pu) : Outport  InitialOutput=0
  wires:
  Break algebraic loop/1 -> Droop/1
  Droop/1 -> Sum/3
  V1meas (pu)/1 -> Product/1, Sum/1
  Ki/1 -> Integrator/1
  Vref (pu)/1 -> Sum/2
  Sum/1 -> Ki/1, Kp/1
  Product/1 -> Break algebraic loop/1
  Kp/1 -> Saturation/1
  Integrator/1 -> Sum1/2
  Saturation/1 -> Sum1/1
  Sum1/1 -> B (pu)/1, Product/2
